simulink model "Noh_Nofusion"  (R2020b)
settings: Solver=FixedStepAuto  StartTime=0.0  StopTime=Inf  FixedStep=0.01  RelTol=1e-3
PostLoadFcn:
  | if any(exist('dsrtsu_mdlpostloadfcn', 'file') ~= 0), dsrtsu_mdlpostloadfcn('Execute', bdroot); end
InitFcn:
  | , if any(exist('rtifpga_mdlclblib', 'file') ~= 0), rtifpga_mdlclblib('Init', bdroot); end,
  | , if any(exist('dsmpb_private', 'file') ~= 0), dsmpb_private('dsmpb_mdlclblib', 'Init', bdroot); end,
undefined symbols (not defined in the file): ACC_TimeGap_DecSetSwt, ACC_TimeGap_IncSetSwt, AccelPedalPosn, AccelPedalPosnVldty, AccelPedlPosnDiagc, AccPedalOverride, ACU_ShiftInProgress, ADAS_Posn_CurLane, AESSwtReq, ALC_SwtReq, BrkPedalSts, CC_ACC_CANCEL_OFFSwt, CC_ACC_CRUISE_OFFSwt, CC_ACC_DecSetSpd_SetSwt, CC_ACC_IncSetSpd_ResuSwt, CC_ACCSwtErr, CharSpd_ms, CSA_NODE, CURRENT_GEAR, CurrentGearValid, DiscIntNeverNeededParam, DrvDoorSts, DrvSBR, DrvTrqReqOvld, ECMACCInterface, ECMRespACC, ELKSwtReq, EngLimpHomeSts, EngSpd, EngState, EngState_PHEV, EngTrqMaxActSpd, EngTrqMinAct, EPS_DrvInpTrqVal_HighReslolution, EPS_FailSts, EPS_LKATorqOvrlDlvd, EPS_LKATorqOvrlDlvdVld, EPS_LKATrqOvlDlvdSts, EPS_SteerMod, EPS_TrqSnsrSts, EQ4_APPINFO, EQ4_LA_ELEM, EQ4_LA_HDR, EQ4_LAP_ELEM, EQ4_LAP_HDR, EQ4_LH_ELEM, EQ4_LH_HDR, EQ4_LRE_ELEM, EQ4_LRE_HDR, ESS_PedSwtReq, ESS_VehSwtReq, FFogLmpSts_F_Pbox, FLWheelDriveDirection, FLWheelSpd, FrntWiprSwtSts, FrntWshrSwtSts, FRWheelDriveDirection, FRWheelSpd, HazardLmpSwtSts, HCU_AccelPedalPosn_Diag ... (+153)
libraries: simulink x132, dsmpblib x27
(part 9 of 14)

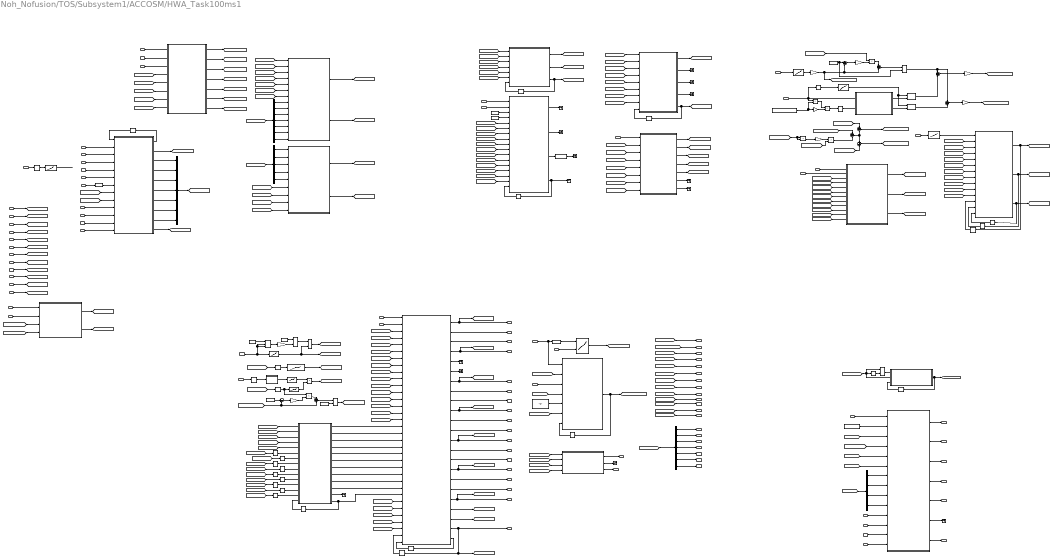
== system Noh_Nofusion/TOS/Subsystem1/ACCOSM/HWA_Task100ms1 ==
  note: EIA
  note: ASI_CalcPreOSF
  note: PLA
  note: ATS
  note: OTL
  ObjRange_m : Inport
  ObjDx_m : Inport  Port=2
  ObjDy_m : Inport  Port=3
  ObjValid : Inport  Port=4
  ObjClassification : Inport  Port=5
  ObjVxG_ms : Inport  Port=6
  ObjVyG_ms : Inport  Port=7
  ObjArG_ms2 : Inport  Port=8
  ObjWidth_m : Inport  Port=9
  ObjCnt : Inport  Port=10
  ObjMoveSts : Inport  Port=11
  ObjBrakeLightIndic : Inport  Port=12
  A2 : Inport  Port=13
  A1 : Inport  Port=14
  Conf : Inport  Port=15
  TimeGap : Inport  Port=16
  ACCMode : Inport  Port=17
  VxvRef_ms : Inport  Port=18
  kapCurvTraj : Inport  Port=19
  AlpSideSlipAngle : Inport  Port=20
  AlpWheelAngle : Inport  Port=21
  alpSumSlideCurveness : Inport  Port=22
  LongitudeAcc : Inport  Port=23
  TarLineValid : Inport  Port=24
  TarLine_A2 : Inport  Port=25
  TarLine_A1 : Inport  Port=26
  TarLine_A0 : Inport  Port=27
  1-D Lookup Table1 : Lookup_n-D  NumberOfTableDimensions=1  BreakpointsForDimension1=[0,8,23,55,60]  Table=[80,80,120,200,200]  RndMeth=Simplest  InputSameDT=on
  1-D Lookup Table2 : Lookup_n-D  NumberOfTableDimensions=1  BreakpointsForDimension1=[0,0.035,0.057,0.1]  Table=[1,1,0,0]  RndMeth=Simplest  InputSameDT=on
  ACCMode1 : InportShadow  Port=17
  ACC_DisplayBar : MATLAB Function  TreatAsAtomicUnit=on
  Abs : Abs
  Abs1 : Abs
  Abs2 : Abs
  AlpSideSlipAngle_1 : InportShadow  Port=20
  Bus Creator : BusCreator  Inputs=7
  Bus Selector : BusSelector  OutputSignals=dxC0,aPC0,bPC0,cPC0,aPC1,bPC1,cPC1
  Bus Selector1 : BusSelector  OutputSignals=dxC0,aPC0,bPC0,aPC1,bPC1
  Bus Selector2 : BusSelector  OutputSignals=dxC0,aPC0,bPC0,cPC0,aPC1,bPC1,cPC1
  Bus Selector3 : BusSelector  OutputSignals=dDeltaX,dDeltaY,CosOfPsi,SinOfPsi
  Compare To Constant : simulink/Logic and Bit Operations/Compare To Constant  relop=>=  const=1  OutDataTypeStr=boolean
  Compare To Constant1 : simulink/Logic and Bit Operations/Compare To Constant  relop=>=  const=0.7  OutDataTypeStr=boolean
  Constant : Constant  Value=15  OutDataTypeStr=single
  Constant1 : Constant  Value=0.6  OutDataTypeStr=single
  Constant3 : Constant  Value=[0.6,0.75,0.9;0.58,0.68,0.77;0.41,0.55,0.63;0.38,0.44,0.49]  OutDataTypeStr=single
  Constant6 : Constant  Value=0.1  OutDataTypeStr=single
  Data Type Conversion7 : DataTypeConversion  OutDataTypeStr=single
  DeltaDx : Lookup_n-D  NumberOfTableDimensions=1  BreakpointsForDimension1=[0,30,60,100,120,130]  Table=[2,4,6,8,9,9]  RndMeth=Simplest  InputSameDT=on
  DeltaDy : Lookup_n-D  NumberOfTableDimensions=1  BreakpointsForDimension1=[0,30,60,100,120,130]  Table=[0.5,0.5,1,1.2,1.5,1.5]  RndMeth=Simplest  InputSameDT=on
  DesireDistance : Lookup_n-D  BreakpointsForDimension1=[1,2,3,4]  BreakpointsForDimension2=[0,2.6,17,25,35,60]  BreakpointsForDimension1DataTypeStr=single  BreakpointsForDimension2DataTypeStr=single  Table=reshape([4,4.3,4.6,4.9,7.8,8.5,9,9.5,18,23,28,34,27,37,47,54,35,49,63,71,60,70,80,85],4,6)  TableDataTypeStr=single  RndMeth=Simplest
      settings: InputPortMap=u0,u1
  Dyc : MATLAB Function  TreatAsAtomicUnit=on
  DycCutIn : MATLAB Function  TreatAsAtomicUnit=on
  DycHistCalc : MATLAB Function  TreatAsAtomicUnit=on
  Fac : Lookup_n-D  NumberOfTableDimensions=1  BreakpointsForDimension1=[0,0.4,0.6,0.8]  Table=[1,1,1.5,1.5]  RndMeth=Simplest  InputSameDT=on
  Gain{,1,3..4} (4 alike) : Gain  Gain=0.5
  Gain2 : Gain  Gain=0.95
  Gain5 : Gain  Gain=0.02
  Gain6 : Gain  Gain=0.95
  Gain8 : Gain  Gain=0.02
  LostTargetCalc : MATLAB Function  TreatAsAtomicUnit=on
  Lpb : MATLAB Function  TreatAsAtomicUnit=on
  Memory{1..2,4,6,13..14} (6 alike) : Memory  InitialCondition=single(zeros(15,1))  InheritSampleTime=on
  Memory10 : Memory  InitialCondition=uint8(0)  InheritSampleTime=on
  Memory12 : Memory  InheritSampleTime=on
  Memory{8,15..16,18..22,25,27..28} (11 alike) : Memory  InitialCondition=single(0)  InheritSampleTime=on
  Memory17 : Memory  InitialCondition=uint8(0)  InheritSampleTime=on
  Memory24 : Memory  InitialCondition=false  InheritSampleTime=on
  Memory26 : Memory  InitialCondition=false  InheritSampleTime=on
  Memory3 : Memory  InheritSampleTime=on
  Memory30 : Memory  InitialCondition=uint8(0)  InheritSampleTime=on
  MinMax : MinMax  Function=max  Inputs=2
  MinMax1 : MinMax  Function=max  Inputs=2
  MinMax2 : MinMax  Inputs=2
  MinMax4 : MinMax  Inputs=2
  MinMax5 : MinMax  Function=max  Inputs=2
  MinMax6 : MinMax  Inputs=2
  OTL1 : Subsystem
  Plaus : MATLAB Function  TreatAsAtomicUnit=on
  Product{,1..6} (7 alike) : Product
  Product7 : Product  Inputs=/**
  Relational Operator1 : RelationalOperator  Operator===  OutDataTypeStr=boolean  RndMeth=Nearest
  Spw : MATLAB Function  TreatAsAtomicUnit=on
  Std : MATLAB Function  TreatAsAtomicUnit=on
  Sum1 : Sum  Inputs=|+-
  Sum10 : Sum  Inputs=-+
  Sum11 : Sum  Inputs=|+-
  Sum{2..4,13} (4 alike) : Sum
  Sum8 : Sum  Inputs=+-
  Sum9 : Sum  Inputs=+-
  Tapped Delay : simulink/Discrete/Tapped Delay  vinit=0.0  samptime=-1  NumDelays=4  DelayOrder=Newest  includeCurrent=on
  TarLineValid1 : InportShadow  Port=24
  TarLine_A0_1 : InportShadow  Port=27
  TarLine_A1_1 : InportShadow  Port=26
  TarLine_A2_1 : InportShadow  Port=25
  TargetBrake : MATLAB Function  TreatAsAtomicUnit=on
  TargetSelect : MATLAB Function  TreatAsAtomicUnit=on
  Terminator{,1,3,9..15,17..20} (14 alike) : Terminator
  TimeCalc : MATLAB Function  TreatAsAtomicUnit=on
  Trajectory : Subsystem  TreatAsAtomicUnit=on
  VxVy : Subsystem
  VxvRef_ms_{1..10} (10 alike) : InportShadow  Port=18
  VycCalc : MATLAB Function  TreatAsAtomicUnit=on
  alpSumSlideCurveness1 : InportShadow  Port=22
  dxMaxFollowPO : Lookup_n-D  NumberOfTableDimensions=1  BreakpointsForDimension1=[8.33,22.22,37.5]  Table=[90,120,120]  InternalRulePriority=Speed  RndMeth=Simplest  InputSameDT=on
  dyLaneWidthMin : Lookup_n-D  NumberOfTableDimensions=1  BreakpointsForDimension1=[0,2.78,8.33,10]  Table=[3,3,2.8,2.8]  InternalRulePriority=Speed  RndMeth=Simplest  InputSameDT=on
  dyLaneWidthMinHalfStatObj1 : Constant  Value=P_Global_DxvFrontBumper_m  OutDataTypeStr=single
  dyLaneWidthMinHalfStatObj10 : Constant  Value=2.2  OutDataTypeStr=single
  dyLaneWidthMinHalfStatObj2 : Constant  Value=2.2  OutDataTypeStr=single
  dyLaneWidthMinHalfStatObj5 : Constant  Value=0  OutDataTypeStr=single
  dyLaneWidthMinHalfStatObj7 : Constant  Value=0  OutDataTypeStr=single
  dyLaneWidthMinHalfStatObj9 : Constant  Value=2.2  OutDataTypeStr=single
  dyLaneWidthSteerAdapt : MATLAB Function  TreatAsAtomicUnit=on
  kapCurvTraj_{1..4} (4 alike) : InportShadow  Port=19
  t_dyLaneWidthSteerAdapt : Lookup_n-D  NumberOfTableDimensions=1  BreakpointsForDimension1=[0,0.02,0.05,0.1]  Table=[0,0,0.7,0.7]  InternalRulePriority=Speed  RndMeth=Simplest  InputSameDT=on
  wCutInVy : MATLAB Function  TreatAsAtomicUnit=on
  wCutOutVy : MATLAB Function  TreatAsAtomicUnit=on
  P0ID : Outport
  P2ID : Outport  Port=2
  P3ID : Outport  Port=3
  TargetBrake_b : Outport  Port=4
  P0Range : Outport  Port=5
  P0Vr : Outport  Port=6
  P2Vr : Outport  Port=7
  P3Vr : Outport  Port=8
  P0ArG : Outport  Port=9
  P2ArG : Outport  Port=10
  P3ArG : Outport  Port=11
  P0Dx : Outport  Port=12
  P2Dx : Outport  Port=13
  P3Dx : Outport  Port=14
  P0Dy : Outport  Port=15
  P2Dy : Outport  Port=16
  P3Dy : Outport  Port=17
  CutIn_b : Outport  Port=18
  TargetExist : Outport  Port=19
  DesireDis : Outport  Port=20
  Signal_ACC_TgtObjBarDisp : Outport  Port=21
  ObjDyc_m : Outport  Port=22
  ObjVy_ms : Outport  Port=23
  ObjVyc_ms : Outport  Port=24
  ObjSpw : Outport  Port=25
  ObjSpwLeft : Outport  Port=26
  ObjSpwRight : Outport  Port=27
  ObjPlaus : Outport  Port=28
  ObjPlausLeft : Outport  Port=29
  ObjPlausRight : Outport  Port=30
  ObjDycHist : Outport  Port=31
  ObjqDycHist : Outport  Port=32
  dxC0 : Outport  Port=33
  aPC0 : Outport  Port=34
  bPC0 : Outport  Port=35
  cPC0 : Outport  Port=36
  aPC1 : Outport  Port=37
  bPC1 : Outport  Port=38
  cPC1 : Outport  Port=39
  OTLValid : Outport  Port=40
  aOTL : Outport  Port=41
  bOTL : Outport  Port=42
  cOTL : Outport  Port=43
  dOTL : Outport  Port=44
  dxMaxOTL : Outport  Port=45
  TargetVyG : Outport  Port=46
  wires:
  TarLine_A0_1/1 -> OTL1/14(TarLineA0)
  TarLineValid1/1 -> OTL1/11(TarLineValid)
  TarLine_A1_1/1 -> OTL1/13(TarLineA1)
  TarLine_A2_1/1 -> OTL1/12(TarLineA2)
  Dyc/10(ObjDyc) -> [ObjDyc_m]
  DesireDistance/1 -> [DesireDistanceChar]
  Memory10/1 -> ACC_DisplayBar/7(DisplayBarK1)
  Constant3/1 -> ACC_DisplayBar/5(Scale)
  ACC_DisplayBar/1(DisplayBar) -> [Signal_ACC_TgtObjBarDisp], Memory10/1
  [TargetRange] -> ACC_DisplayBar/4(TargetRange)
  [TargetExist] -> ACC_DisplayBar/6(TargetExist)
  ACCMode/1 -> ACC_DisplayBar/3(ACCmode)
  TimeGap/1 -> ACC_DisplayBar/1(TimeGap), Data Type Conversion7/1
  VxvRef_ms_3/1 -> dyLaneWidthMin/1
  dyLaneWidthMin/1 -> Gain/1
  Gain/1 -> [dyLaneWidthMinHalf], Sum2/2, Sum1/2  "dyLaneWidthMinHalf"
  dyLaneWidthMinHalfStatObj1/1 -> Product/2, Gain3/1
  kapCurvTraj/1 -> Abs1/1, Product/1, dyLaneWidthSteerAdapt/1(kap)
  Product/1 -> Product1/1
  Gain3/1 -> Product1/2
  Product1/1 -> Abs/1
  Abs/1 -> dyLaneWidthSteerAdapt/2(dyAdapt)  "dyAdapt"
  Abs1/1 -> t_dyLaneWidthSteerAdapt/1
  t_dyLaneWidthSteerAdapt/1 -> MinMax1/1, MinMax/1
  dyLaneWidthSteerAdapt/1(dyLaneAdaptLeft) -> MinMax/2
  dyLaneWidthSteerAdapt/2(dyLaneAdaptRight) -> MinMax1/2
  MinMax/1 -> Sum3/2  "dyLaneWidthSteerAdaptLeft"
  MinMax1/1 -> Sum4/2  "dyLaneWidthSteerAdaptRight"
  Sum1/1 -> Gain5/1
  Gain5/1 -> Product2/2
  [ObjDx_m] -> Product2/1
  Product2/1 -> Sum2/1
  Sum2/1 -> MinMax2/1
  dyLaneWidthMinHalfStatObj2/1 -> MinMax2/2, Sum1/1
  MinMax2/1 -> Sum3/1, Sum4/1
  Sum3/1 -> Gain2/1
  VxvRef_ms_5/1 -> VxVy/1(VxvRef)
  VxVy/1(Vx) -> [ObjVx_ms]
  VxVy/2(Vy) -> [ObjVy_ms]
  [ObjVyG_ms] -> VxVy/4(VyG)
  [ObjVxG_ms] -> VxVy/3(VxG)
  kapCurvTraj_3/1 -> VxVy/2(Kap)
  kapCurvTraj_2/1 -> Trajectory/1(Kap)
  AlpSideSlipAngle/1 -> Trajectory/3(AlpSideSlipAngle)
  VxvRef_ms_6/1 -> Trajectory/2(VxvRef)
  [ObjValid] -> Trajectory/4(ObjValid)
  [ObjCnt] -> Trajectory/8(ObjCntAlive)
  [ObjDx_m] -> Trajectory/5(ObjDx)
  [ObjDy_m] -> Trajectory/6(ObjDy)
  [ObjMoveSts] -> Trajectory/7(ObjClass)
  Memory8/1 -> Dyc/1(kapTrajFiltK1)
  Dyc/1(kapTrajFilt) -> Memory8/1
  AlpSideSlipAngle_1/1 -> Dyc/4(alpSideSlipAngle)
  kapCurvTraj_1/1 -> Dyc/3(kapTraj)
  ObjDx_m/1 -> [ObjDx_m]
  Compare To Constant/1 -> Dyc/7(LineValid)
  VxvRef_ms_7/1 -> Dyc/2(vRef)
  1-D Lookup Table2/1 -> ?  "AlpWheelAngleFactor"
  Abs2/1 -> 1-D Lookup Table2/1
  AlpWheelAngle/1 -> Abs2/1
  ObjRange_m/1 -> [ObjRange_m]
  ObjMoveSts/1 -> [ObjMoveSts]
  ObjVxG_ms/1 -> [ObjVxG_ms]
  ObjWidth_m/1 -> [ObjWidth_m]
  ObjClassification/1 -> [ObjClassification]
  ObjArG_ms2/1 -> [ObjArG_ms2]
  Conf/1 -> Compare To Constant/1
  ObjDy_m/1 -> [ObjDy_m]
  ObjCnt/1 -> [ObjCnt]
  ObjVyG_ms/1 -> [ObjVyG_ms]
  [ObjDy_m] -> Dyc/9(ObjDy)
  [ObjDx_m] -> Dyc/8(ObjDx)
  Dyc/9(cPC1) -> Bus Creator/7
  Dyc/7(aPC1) -> Bus Creator/5
  Dyc/8(bPC1) -> Bus Creator/6
  ObjValid/1 -> [ObjValid]
  Dyc/4(aPC0) -> Bus Creator/2
  Dyc/5(bPC0) -> Bus Creator/3
  Dyc/6(cPC0) -> Bus Creator/4
  Dyc/3(dxC0) -> Bus Creator/1
  Data Type Conversion7/1 -> DesireDistance/1
  Sum4/1 -> Gain6/1
  Bus Creator/1 -> [EgoLine]
  [ObjValid] -> DycHistCalc/7(ObjValid)
  DycHistCalc/1(ObjDycHist) -> [ObjDycHist]
  DycHistCalc/2(ObjqDycHist) -> [ObjqDycHist]
  [ObjValid] -> VycCalc/6(ObjValid)
  [ObjDx_m] -> VycCalc/7(ObjDx)
  [ObjVxG_ms] -> VycCalc/8(ObjVxG)
  [ObjVyG_ms] -> VycCalc/9(ObjVyG)
  VycCalc/1(ObjVyc) -> [ObjVyc]
  [EgoLine] -> Bus Selector/1
  Bus Selector/4 -> DycHistCalc/11(cP0)  "<cPC0>"
  Bus Selector/3 -> DycHistCalc/10(bP0)  "<bPC0>"
  Bus Selector/5 -> DycHistCalc/12(aP1)  "<aPC1>"
  Bus Selector/2 -> DycHistCalc/9(aP0)  "<aPC0>"
  Bus Selector/6 -> DycHistCalc/13(bP1)  "<bPC1>"
  Bus Selector/1 -> DycHistCalc/8(dxC0)  "<dxC0>"
  Bus Selector/7 -> DycHistCalc/14(cP1)  "<cPC1>"
  [EgoLine] -> Bus Selector1/1
  Bus Selector1/3 -> VycCalc/3(bP0)  "<bPC0>"
  Bus Selector1/2 -> VycCalc/2(aP0)  "<aPC0>"
  Bus Selector1/4 -> VycCalc/4(aP1)  "<aPC1>"
  Bus Selector1/1 -> VycCalc/1(dxC0)  "<dxC0>"
  Bus Selector1/5 -> VycCalc/5(bP1)  "<bPC1>"
  Dyc/2(kapCourseErr) -> [kapCourseErr]
  [ObjDx_m] -> Product3/2, Product3/1
  Product3/1 -> Gain4/1
  Gain4/1 -> Product4/1
  [kapCourseErr] -> Product4/2
  Product4/1 -> Sum8/2
  [dyLaneWidthMinHalf] -> Sum8/1
  [dyLaneWidthRight] -> Sum9/1
  Sum8/1 -> Sum9/2, Sum10/1
  Sum9/1 -> [dyEdgeWidthRight]  "dyEdgeWidthRight"
  [dyLaneWidthLeft] -> Sum10/2
  Sum10/1 -> [dyEdgeWidthLeft]  "dyEdgeWidthLeft"
  VycCalc/2(ObjYawAngle) -> [ObjYawAngle]
  VxvRef_ms_1/1 -> Lpb/1(vRef)
  alpSumSlideCurveness/1 -> Lpb/2(alpSumSlideCurveness)
  [ObjValid] -> Lpb/3(ObjValid)
  [ObjDyc_m] -> Lpb/4(ObjDyc)
  [ObjDycHist] -> Lpb/5(ObjDycHist)
  [ObjqDycHist] -> Lpb/6(ObjqDycHist)
  [ObjVyc] -> Lpb/7(ObjVyc)
  [ObjYawAngle] -> Lpb/8(ObjYawAngle)
  Lpb/1(ObjLpb) -> [ObjLpb]
  Lpb/2(ObjLpbL) -> [ObjLpbLeft]
  Lpb/3(ObjLpbR) -> [ObjLpbRight]
  [dyLaneWidthRight] -> Lpb/9(ObjDylaneEdgeRight)
  [dyEdgeWidthLeft] -> Lpb/12(ObjDyEdgeWidthLeft)
  [dyEdgeWidthRight] -> Lpb/10(ObjDyEdgeWidthRight)
  [dyLaneWidthLeft] -> Lpb/11(ObjDylaneEdgeLeft)
  [ObjValid] -> DycCutIn/1(ObjValid)
  [ObjDyc_m] -> DycCutIn/2(ObjDyc)
  [ObjMoveSts] -> DycCutIn/3(ObjMoveSts)
  [ObjCnt] -> DycCutIn/4(ObjCnt)
  [ObjDycHist] -> DycCutIn/5(ObjDycHist)
  [ObjqDycHist] -> DycCutIn/6(ObjqDycHist)
  DycCutIn/3(ObjDycFilt) -> [ObjDycFilt], Memory1/1
  DycCutIn/1(ObjDycCutIn) -> [ObjDycCutIn]
  Memory1/1 -> DycCutIn/7(dycFiltK1)
  DycCutIn/2(ObjMove_b) -> [ObjDrive_b]
  [ObjValid] -> wCutOutVy/5(ObjValid)
  [ObjDycCutIn] -> wCutOutVy/6(ObjDycCutIn)
  [ObjWidth_m] -> wCutOutVy/7(ObjWidth)
  [ObjVyc] -> wCutOutVy/8(ObjVyc)
  [ObjDx_m] -> wCutOutVy/9(ObjDx)
  [ObjDycFilt] -> wCutOutVy/16(ObjDycFilt)
  wCutOutVy/4(ObjwCutoutVy) -> Terminator17/1, Memory2/1
  Memory2/1 -> wCutOutVy/17(ObjwCutoutVyK1)
  wCutOutVy/1(ObjtPrediction4CutOut) -> Terminator14/1
  wCutOutVy/2(ObjDycCutOutPredict) -> Terminator15/1
  kapCurvTraj_4/1 -> wCutOutVy/2(kap)
  VxvRef_ms_8/1 -> wCutOutVy/1(vRef)
  dyLaneWidthMinHalfStatObj5/1 -> wCutOutVy/3(tDirIndLeft)
  dyLaneWidthMinHalfStatObj7/1 -> wCutOutVy/4(tDirIndRight)
  [ObjDy_m] -> wCutOutVy/10(ObjDy)
  [ObjVx_ms] -> wCutOutVy/11(ObjVx)
  [ObjVy_ms] -> wCutOutVy/12(ObjVy)
  [ObjDyc_m] -> wCutOutVy/13(ObjDyc)
  [ObjDrive_b] -> wCutOutVy/14(ObjDrive_b)
  [ObjCnt] -> wCutOutVy/15(ObjCnt)
  wCutOutVy/3(ObjwCutOutTurnOff) -> Compare To Constant1/1
  [ObjValid] -> wCutInVy/1(ObjValid)
  [ObjDycCutIn] -> wCutInVy/2(ObjDycCutIn)
  [ObjWidth_m] -> wCutInVy/3(ObjWidth)
  [ObjVyc] -> wCutInVy/4(ObjVyc)
  [ObjDx_m] -> wCutInVy/5(ObjDx)
  [ObjDy_m] -> wCutInVy/6(ObjDy)
  [ObjCnt] -> wCutInVy/7(ObjCnt)
  [ObjDycFilt] -> wCutInVy/8(ObjDycFilt)
  wCutInVy/5(ObjwCutInVy) -> [ObjwCutIn], Memory4/1
  Memory4/1 -> wCutInVy/9(ObjwCutInVyK1)
  wCutInVy/2(ObjtPrediction4CutIn) -> Terminator18/1
  wCutInVy/3(ObjDycCutInPredict) -> Terminator19/1
  wCutInVy/1(DycASI) -> [DycASI]
  alpSumSlideCurveness1/1 -> Spw/1(AlpSumSlideCurveness)
  [kapCourseErr] -> Spw/2(kapCourseErr)
  [ObjValid] -> Spw/3(ObjValid)
  [DycASI] -> Spw/4(DycASI)
  [ObjDx_m] -> Spw/5(ObjDx)
  Spw/1(ObjSpw) -> [ObjSpw]
  Spw/2(ObjSpwLeft) -> [ObjSpwLeft]
  Spw/3(ObjSpwRight) -> [ObjSpwRight]
  wCutInVy/4(ObjCutIn_b) -> Terminator20/1
  Spw/4(ObjOnLeft) -> [ObjOnLeft]
  Spw/5(ObjOnRight) -> [ObjOnRight]
  [ObjDyc_m] -> Spw/6(ObjDyc)
  [ObjDycHist] -> Spw/7(ObjDycHist)
  [ObjqDycHist] -> Spw/8(ObjqDycHist)
  Plaus/3(ObjPlausRight) -> Memory6/1, [ObjPlausRight]
  Plaus/2(ObjPlausLeft) -> [ObjPlausLeft], Memory13/1
  Plaus/1(ObjPlaus) -> [ObjPlaus], Memory14/1
  dxMaxFollowPO/1 -> Plaus/1(dxMaxFollow)
  VxvRef_ms_9/1 -> dxMaxFollowPO/1
  [ObjValid] -> Plaus/2(ObjValid)
  [ObjDx_m] -> Plaus/3(ObjDx)
  [ObjVx_ms] -> Plaus/4(ObjVx)
  [ObjOnLeft] -> Plaus/5(ObjOnLeft)
  [ObjOnRight] -> Plaus/6(ObjOnRight)
  [ObjDycHist] -> Plaus/7(ObjDycHist)
  [ObjqDycHist] -> Plaus/8(ObjqDycHist)
  [ObjLpb] -> Plaus/9(ObjLpb)
  [ObjLpbLeft] -> Plaus/10(ObjLpbLeft)
  [ObjLpbRight] -> Plaus/11(ObjLpbRight)
  Memory6/1 -> Plaus/14(ObjPlausRightK1)
  Memory13/1 -> Plaus/13(ObjPlausLeftK1)
  Memory14/1 -> Plaus/12(ObjPlausK1)
  [ObjDx_m] -> TargetSelect/6(Dx)
  TargetSelect/12(P3ArG) -> P3ArG/1
  TargetSelect/9(P3Vr) -> P3Vr/1
  [ObjDyc_m] -> ObjDyc_m/1
  TargetSelect/17(P2Dy) -> P2Dy/1
  TargetSelect/11(P2ArG) -> P2ArG/1
  [ObjMoveSts] -> TargetSelect/30(MoveSts)
  [ObjArG_ms2] -> TargetSelect/8(ArG)
  TargetSelect/18(P3Dy) -> P3Dy/1
  TargetSelect/8(P2Vr) -> P2Vr/1
  [ObjClassification] -> TargetSelect/29(Classfication)
  [ObjValid] -> TargetSelect/3(Valid)
  TargetSelect/3(P3ID) -> P3ID/1
  VxvRef_ms/1 -> TargetSelect/2(vRef)
  ACCMode1/1 -> TargetSelect/1(ACCmode)
  [TarLimDx] -> TargetSelect/31(TarLimDx)
  Memory24/1 -> TargetSelect/33(TargetExistK1)
  TargetSelect/4(P0Range) -> P0Range/1, [TargetRange]
  TargetSelect/15(P3Dx) -> P3Dx/1
  [ObjRange_m] -> TargetSelect/4(Range)
  [ObjVx_ms] -> TargetSelect/5(Vr)
  [Signal_ACC_TgtObjBarDisp] -> Signal_ACC_TgtObjBarDisp/1
  [ObjSpwRight] -> TargetSelect/16(spwRight)
  TargetSelect/2(P2ID) -> P2ID/1
  [ObjVy_ms] -> ObjVy_ms/1
  [ObjDy_m] -> TargetSelect/7(Dy)
  TargetSelect/13(P0Dx) -> [TargetDx], P0Dx/1
  TargetSelect/7(P0Vr) -> [TargetVr], P0Vr/1
  [DesireDistanceChar] -> DesireDis/1  "DesireDis"
  TargetSelect/19(TargetCutIn_b) -> [TargetCutIn_b], CutIn_b/1
  TargetSelect/22(TargetExist) -> Memory24/1, [TargetExist], TargetExist/1
  TargetSelect/10(P0ArG) -> [TargetArG], P0ArG/1
  TargetSelect/14(P2Dx) -> P2Dx/1
  TargetSelect/16(P0Dy) -> [TargetDy], P0Dy/1
  [ObjPlaus] -> TargetSelect/12(plaus)
  [ObjwCutIn] -> TargetSelect/13(wCutIn)
  [ObjSpw] -> TargetSelect/14(spw)
  [ObjSpwLeft] -> TargetSelect/15(spwLeft)
  MinMax4/1 -> [dyLaneWidth]
  LostTargetCalc/12(tTargetLost) -> Memory27/1, TargetSelect/27(tTargetLost)
  [ObjValid] -> LostTargetCalc/1(ObjValid)
  [ObjDx_m] -> LostTargetCalc/2(ObjDx)
  [ObjDy_m] -> LostTargetCalc/3(ObjDy)
  TargetSelect/20(P0Dyc) -> [TargetDyc]
  TargetSelect/21(P0Vyc) -> [TargetVyc]
  [TargetID] -> Memory17/1
  Memory17/1 -> LostTargetCalc/6(P0IDK1)
  [TargetVr] -> Memory18/1
  Memory18/1 -> LostTargetCalc/7(P0VxK1)
  Memory20/1 -> LostTargetCalc/8(P0DxK1)
  Memory21/1 -> LostTargetCalc/9(P0DyK1)
  Memory22/1 -> LostTargetCalc/12(P0DycK1)
  Memory25/1 -> LostTargetCalc/13(P0VycK1)
  Memory26/1 -> LostTargetCalc/14(P0CutIn_bK1)
  Memory27/1 -> LostTargetCalc/15(tTargetLostK1)
  [TargetDx] -> Memory20/1
  [TargetDy] -> Memory21/1
  [TargetDyc] -> Memory22/1
  [TargetVyc] -> Memory25/1
  [TargetCutIn_b] -> Memory26/1
  [ObjVyc] -> TargetSelect/10(Vyc)
  [ObjDyc_m] -> TargetSelect/9(Dyc)
  dyLaneWidthMinHalfStatObj9/1 -> Sum11/1
  Sum11/1 -> Gain8/1
  Gain8/1 -> Product6/2
  Sum13/1 -> MinMax4/1
  Product6/1 -> Sum13/1
  [dyLaneWidthMinHalf] -> Sum13/2, Sum11/2  "dyLaneWidthMinHalf"
  Memory19/1 -> LostTargetCalc/10(P0RangeK1)
  [TargetRange] -> Memory19/1
  Memory28/1 -> LostTargetCalc/11(P0ArGK1)
  [TargetArG] -> Memory28/1
  Memory15/1 -> Product6/1, DeltaDx/1
  TargetSelect/1(P0ID) -> P0ID/1, [TargetID]
  TargetSelect/23(TargetReplacedCnt) -> Memory30/1
  Memory30/1 -> TargetSelect/34(TargetReplacedCntK1)
  DeltaDy/1 -> [DeltaDy]
  Memory16/1 -> DeltaDy/1
  [TargetDy] -> Memory16/1
  Product5/1 -> [DeltaDx]
  DeltaDx/1 -> Product5/2
  LongitudeAcc/1 -> Tapped Delay/1
  [TargetDx] -> Memory15/1
  Std/1(y) -> Fac/1
  Fac/1 -> Product5/1
  Tapped Delay/1 -> Std/1(u)
  [DesireDistanceChar] -> ACC_DisplayBar/2(DesireDistance)
  [DeltaDx] -> LostTargetCalc/4(DeltaDx)
  [DeltaDy] -> LostTargetCalc/5(DeltaDy)
  dyLaneWidthMinHalfStatObj10/1 -> MinMax4/2
  LostTargetCalc/1(ReID) -> TargetSelect/17(ReID)
  LostTargetCalc/2(ReRange) -> TargetSelect/18(ReRange)
  LostTargetCalc/3(ReArG) -> TargetSelect/19(ReArG)
  LostTargetCalc/4(ReDx) -> TargetSelect/20(ReDx)
  LostTargetCalc/5(ReDy) -> TargetSelect/21(ReDy)
  LostTargetCalc/6(ReVx) -> TargetSelect/22(ReVx)
  LostTargetCalc/7(ReCutIn_b) -> TargetSelect/23(ReCutIn_b)
  LostTargetCalc/8(ReDyc) -> TargetSelect/24(ReDyc)
  LostTargetCalc/9(ReVyc) -> TargetSelect/25(ReVyc)
  LostTargetCalc/10(TargetLost_b) -> TargetSelect/26(TargetLost_b)
  [dyLaneWidth] -> TargetSelect/28(dyLaneWidth)
  LostTargetCalc/11(Covered_b) -> Terminator9/1
  [ObjVyc] -> ObjVyc_ms/1
  [ObjSpw] -> ObjSpw/1
  [ObjSpwLeft] -> ObjSpwLeft/1
  [ObjSpwRight] -> ObjSpwRight/1
  [ObjPlaus] -> ObjPlaus/1
  [ObjPlausLeft] -> ObjPlausLeft/1
  [ObjPlausRight] -> ObjPlausRight/1
  TargetSelect/5(P2Range) -> Terminator10/1
  TargetSelect/6(P3Range) -> Terminator11/1
  [EgoLine] -> Bus Selector2/1
  Bus Selector2/1 -> dxC0/1  "<dxC0>"
  Bus Selector2/2 -> aPC0/1  "<aPC0>"
  Bus Selector2/3 -> bPC0/1  "<bPC0>"
  Bus Selector2/4 -> cPC0/1  "<cPC0>"
  Bus Selector2/5 -> aPC1/1  "<aPC1>"
  Bus Selector2/6 -> bPC1/1  "<bPC1>"
  Bus Selector2/7 -> cPC1/1  "<cPC1>"
  Spw/6(ObjDycASI) -> Terminator12/1
  Spw/7(ObjDyKapErr) -> Terminator13/1
  [ObjqDycHist] -> ObjqDycHist/1
  [ObjDycHist] -> ObjDycHist/1
  A2/1 -> Dyc/5(A2)
  A1/1 -> Dyc/6(A1)
  [TargetID] -> TargetBrake/1(ID)
  [ObjBrakeLightIndic] -> TargetBrake/4(BrakeLightIndic)
  ObjBrakeLightIndic/1 -> [ObjBrakeLightIndic]
  TargetBrake/1(TargetBrake_b) -> TargetBrake_b/1
  VxvRef_ms_2/1 -> DesireDistance/2
  Constant/1 -> MinMax5/1
  VxvRef_ms_4/1 -> Product7/2, Product7/3, 1-D Lookup Table1/1
  1-D Lookup Table1/1 -> MinMax6/2, [TarLimDx]
  Gain1/1 -> MinMax5/2
  Product7/1 -> Gain1/1
  MinMax5/1 -> MinMax6/1
  [TarLimS0Dx] -> TargetSelect/32(TarLimS0Dx)
  Constant1/1 -> Product7/1
  MinMax6/1 -> [TarLimS0Dx]
  [ObjCnt] -> TargetSelect/11(Cnt)
  Trajectory/1(Out8) -> [TrajHistBufferBTrajEnd]
  Trajectory/2(Out9) -> [ObjTrajNumber]
  Trajectory/3(Out10) -> [TrajCurrentIndex]
  Trajectory/4(Out11) -> [TrajHistBufferBValid]
  Trajectory/5(Out12) -> [TrajHistBufferDxv]
  Trajectory/6(Out13) -> [TrajHistBufferDyv]
  [TrajHistBufferBTrajEnd] -> DycHistCalc/1(TrajHistBufferBTrajEnd)
  [ObjTrajNumber] -> DycHistCalc/2(ObjTrajNumber)
  [TrajCurrentIndex] -> DycHistCalc/3(TrajCurrentIndex)
  [TrajHistBufferBValid] -> DycHistCalc/4(TrajHistBufferBValid)
  [TrajHistBufferDxv] -> DycHistCalc/5(TrajHistBufferDxv)
  [TrajHistBufferDyv] -> DycHistCalc/6(TrajHistBufferDyv)
  TarLine_A1/1 -> Dyc/12(TarLineA1)
  TarLineValid/1 -> Dyc/10(TarLineValid)
  TarLine_A2/1 -> Dyc/11(TarLineA2)
  Compare To Constant1/1 -> Terminator1/1
  [ObjVyG_ms] -> TargetBrake/3(VyG)
  TargetBrake/3(TargetVyG) -> TargetVyG/1
  [ObjVxG_ms] -> TargetBrake/2(VxG)
  TargetBrake/2(TargetVxG) -> Terminator3/1
  [TargetID] -> TimeCalc/2(TargetID), Relational Operator1/1, Memory12/1
  Relational Operator1/1 -> TimeCalc/1(SameTarget)
  TimeCalc/1(tSameHandleT) -> Memory3/1, [tSameHandleT1]
  Memory3/1 -> TimeCalc/3(tSameHandleTK1)
  Memory12/1 -> Relational Operator1/2
  Trajectory/7(EgoMove) -> [EgoMove]
  Constant6/1 -> OTL1/2(tCycle)
  Bus Selector3/2 -> OTL1/8(EgoDDeltaY)  "<dDeltaY>"
  Bus Selector3/4 -> OTL1/10(EgoSinOfPsi)  "<SinOfPsi>"
  [TargetDy] -> OTL1/6(P0Dy)
  [tSameHandleT1] -> OTL1/3(tSameHandle)
  Bus Selector3/3 -> OTL1/9(EgoCosOfPsi)  "<CosOfPsi>"
  Bus Selector3/1 -> OTL1/7(EgoDDeltaX)  "<dDeltaX>"
  [TargetDx] -> OTL1/5(P0Dx)
  [EgoMove] -> Bus Selector3/1
  OTL1/1(LineValid) -> OTLValid/1
  OTL1/2(a) -> aOTL/1
  OTL1/3(b) -> bOTL/1
  OTL1/4(c) -> cOTL/1
  OTL1/5(d) -> dOTL/1
  OTL1/7(dxMax) -> dxMaxOTL/1
  OTL1/6(dxMin) -> Terminator/1
  TarLine_A0/1 -> Dyc/13(TarLineA0)
  Gain2/1 -> [dyLaneWidthLeft]
  Gain6/1 -> [dyLaneWidthRight]
  [TargetCutIn_b] -> OTL1/4(CutIn)
  VxvRef_ms_10/1 -> OTL1/1(vRef)

== system Noh_Nofusion/TOS/Subsystem1/ACCOSM/ObjMatrixTransit ==
  EQ4_OBJ : Inport
  Bus Creator : BusCreator  Inputs=14
  Bus Selector4 : BusSelector  OutputSignals=EQ4_OBJ_HDR.OBJ_Sync_ID,EQ4_OBJ_HDR.OBJ_VRU_Count,EQ4_OBJ_HDR.OBJ_VD_Count,EQ4_OBJ_HDR.OBJ_General_OBJ_Count,EQ4_OBJ_HDR.OBJ_Animal_Count,EQ4_OBJ_ELEM
  Data Type Conversion : DataTypeConversion
  IFV2FrontBumper : Constant  Value=1.7  OutDataTypeStr=single
  IFV2RearAxis : Constant  Value=2.1  OutDataTypeStr=single
  Subsystem : Subsystem
  Sum : Sum  Inputs=++++
  Sum1 : Sum  Inputs=|-+
  Sum5 : Sum  Inputs=++|
  Terminator1 : Terminator
  VisObjSts : Outport
  wires:
  Subsystem/6(ObjLatVel) -> Bus Creator/7  "ObjLatVel"
  Subsystem/4(ObjClassification) -> Bus Creator/5  "ObjClassification"
  Subsystem/2(ObjValid) -> Bus Creator/3  "ObjValid"
  Subsystem/7(ObjLongAccel) -> Bus Creator/8  "ObjLongAccel"
  Subsystem/5(ObjLatPos) -> Bus Creator/6  "ObjLatPos"
  Subsystem/3(ObjBrakeLightIndic) -> Bus Creator/4  "ObjBrakeLightIndic"
  Subsystem/9(ObjWidth) -> Bus Creator/10  "ObjWidth"
  Subsystem/12(ObjLongPos) -> Sum1/2, Sum5/1
  Subsystem/8(ObjLongVel) -> Bus Creator/9  "ObjLongVel"
  Subsystem/10(ObjCnt) -> Bus Creator/11  "ObjCnt"
  Sum1/1 -> Bus Creator/13  "ObjRange_m"
  Subsystem/11(ObjMoveSts) -> Bus Creator/12  "ObjMoveSts"
  Sum5/1 -> Bus Creator/14  "ObjDx_m"
  IFV2RearAxis/1 -> Sum5/2
  Data Type Conversion/1 -> Bus Creator/1  "Cnt"
  IFV2FrontBumper/1 -> Sum1/1
  Bus Creator/1 -> VisObjSts/1  "ObjSts"
  Subsystem/1(ObjID) -> Bus Creator/2  "ObjID"
  Bus Selector4/6 -> Subsystem/2(<EQ4_OBJ_ELEM>)  "<EQ4_OBJ_ELEM>"
  Sum/1 -> Subsystem/1(Count)
  Bus Selector4/4 -> Sum/3  "<OBJ_General_OBJ_Count>"
  Bus Selector4/3 -> Sum/2  "<OBJ_VD_Count>"
  Bus Selector4/2 -> Sum/1  "<OBJ_VRU_Count>"
  Bus Selector4/1 -> Data Type Conversion/1  "<OBJ_Sync_ID>"
  Bus Selector4/5 -> Sum/4  "<OBJ_Animal_Count>"
  EQ4_OBJ/1 -> Bus Selector4/1
  Subsystem/13(P) -> Terminator1/1

== system Noh_Nofusion/TOS/Subsystem1/ACCOSM/rollingcounter 1 ==
  Constant7 : Constant  OutDataTypeStr=Inherit: Inherit via back propagation
  Constant8 : Constant  Value=7  OutDataTypeStr=Inherit: Inherit via back propagation
  Constant9 : Constant  Value=0  OutDataTypeStr=Inherit: Inherit via back propagation
  Relational Operator : RelationalOperator  Operator=>  OutDataTypeStr=boolean  RndMeth=Nearest
  Sum : Sum  Inputs=|++
  Switch : Switch  Criteria=u2 ~= 0  Threshold=1
  Unit Delay : UnitDelay  SampleTime=-1  HasFrameUpgradeWarning=on
  cnt : Outport
  wires:
  Constant9/1 -> Switch/1
  Sum/1 -> Switch/3, Relational Operator/1
  Constant8/1 -> Relational Operator/2
  Unit Delay/1 -> Sum/2
  Constant7/1 -> Sum/1
  Relational Operator/1 -> Switch/2
  Switch/1 -> cnt/1, Unit Delay/1

== system Noh_Nofusion/Common1/Subsystem7/DS/DriverStsConditnJudge/DSGoodUnbeliv2LowDistractnJudge ==
  note: %Note
      | Conditions of distraction state from Good∥Unbelievable to Low as follow:
      | DMSSts_ACC is 0x02: Active
      | && HeadDetn is 0x01: Yes
      | && DistrctnLevel_ACC is 0x01: Low level distraction
      | && DistrctnQlty_ACC≥ 85%
      | && During time≥1s(adjustable)
  canDMSSts : Inport
  canHeadDetn : Inport  Port=2
  canDistrctnLevel : Inport  Port=3
  canDistrctnQlty : Inport  Port=4
  PtDSGoodUnbeliv2LowDistrctn : Inport  Port=5
  Compare To Constant : simulink/Logic and Bit Operations/Compare To Constant  relop===  const=2  OutDataTypeStr=boolean
  Compare To Constant1 : simulink/Logic and Bit Operations/Compare To Constant  relop===  const=1  OutDataTypeStr=boolean
  Compare To Constant2 : simulink/Logic and Bit Operations/Compare To Constant  relop===  const=1  OutDataTypeStr=boolean
  Compare To Constant4 : simulink/Logic and Bit Operations/Compare To Constant  relop=>=  const=85  OutDataTypeStr=boolean
  Compare To Constant8 : simulink/Logic and Bit Operations/Compare To Constant  relop=<=  const=100  OutDataTypeStr=boolean
  Data Type Conversion : DataTypeConversion  OutDataTypeStr=single
  Logical Operator : Logic  Inputs=5  AllPortsSameDT=off  OutDataTypeStr=boolean
  Relational Operator : RelationalOperator  OutDataTypeStr=boolean  RndMeth=Simplest
  counter : DiscreteIntegrator  ExternalReset=either  SampleTime=-1  LimitOutput=on  UpperSaturationLimit=10  LowerSaturationLimit=-10  ICPrevOutput=DiscIntNeverNeededParam  ICPrevScaledInput=DiscIntNeverNeededParam
  DSGoodUnbeliv2LowDistractn : Outport
  wires:
  Data Type Conversion/1 -> counter/1, counter/2
  PtDSGoodUnbeliv2LowDistrctn/1 -> Relational Operator/2
  Relational Operator/1 -> DSGoodUnbeliv2LowDistractn/1
  Compare To Constant8/1 -> Logical Operator/5
  Compare To Constant4/1 -> Logical Operator/4
  Compare To Constant2/1 -> Logical Operator/3
  Compare To Constant/1 -> Logical Operator/1
  Compare To Constant1/1 -> Logical Operator/2
  canDistrctnQlty/1 -> Compare To Constant4/1, Compare To Constant8/1
  counter/1 -> Relational Operator/1
  Logical Operator/1 -> Data Type Conversion/1
  canDistrctnLevel/1 -> Compare To Constant2/1
  canHeadDetn/1 -> Compare To Constant1/1
  canDMSSts/1 -> Compare To Constant/1

== system Noh_Nofusion/Common1/Subsystem7/DS/DriverStsConditnJudge/DSGoodUnbeliv2LowDrowsnsJudge ==
  note: %Note
      | Conditions of drowsns state from Good∥Unbelievable to Low as follow:
      | DMSSts_ACC is 0x02: Active
      | && HeadDetn is 0x01: Yes
      | && DrowsnsLevel_ACC is 0x1: Low level Drowsiness
      | && DrowsnsQlty_ACC≥85%
      | && During time≥3s(adjustable)
  canDMSSts : Inport
  canHeadDetn : Inport  Port=2
  canDrowsnsLevel : Inport  Port=3
  PtDSGoodUnbeliv2LowDrowsns : Inport  Port=4
  Compare To Constant : simulink/Logic and Bit Operations/Compare To Constant  relop===  const=2  OutDataTypeStr=boolean
  Compare To Constant1 : simulink/Logic and Bit Operations/Compare To Constant  relop===  const=1  OutDataTypeStr=boolean
  Compare To Constant2 : simulink/Logic and Bit Operations/Compare To Constant  relop===  const=1  OutDataTypeStr=boolean
  Data Type Conversion : DataTypeConversion  OutDataTypeStr=single
  Logical Operator : Logic  Inputs=3  AllPortsSameDT=off  OutDataTypeStr=boolean
  Relational Operator : RelationalOperator  OutDataTypeStr=boolean  RndMeth=Simplest
  counter : DiscreteIntegrator  ExternalReset=either  SampleTime=-1  LimitOutput=on  UpperSaturationLimit=10  LowerSaturationLimit=-10  ICPrevOutput=DiscIntNeverNeededParam  ICPrevScaledInput=DiscIntNeverNeededParam
  DSGoodUnbeliv2LowDrowsns : Outport
  wires:
  Data Type Conversion/1 -> counter/2, counter/1
  PtDSGoodUnbeliv2LowDrowsns/1 -> Relational Operator/2
  canDMSSts/1 -> Compare To Constant/1
  canHeadDetn/1 -> Compare To Constant1/1
  canDrowsnsLevel/1 -> Compare To Constant2/1
  Logical Operator/1 -> Data Type Conversion/1
  counter/1 -> Relational Operator/1
  Compare To Constant1/1 -> Logical Operator/2
  Compare To Constant/1 -> Logical Operator/1
  Compare To Constant2/1 -> Logical Operator/3
  Relational Operator/1 -> DSGoodUnbeliv2LowDrowsns/1

== system Noh_Nofusion/Common1/Subsystem7/DS/DriverStsConditnJudge/DSGoodUnbeliv2MidDistractnJudge ==
  note: %Note
      | Conditions of distraction state from Good∥Unbelievable to Middle as follow:
      | DMSSts_ACC is 0x02: Active
      | && HeadDetn is 0x01: Yes
      | && DistrctnLevel_ACC is 0x02: Middle level distraction
      | && DistrctnQlty_ACC≥ 85%
      | && During time≥2s(adjustable)
  canDMSSts : Inport
  canHeadDetn : Inport  Port=2
  canDistrctnLevel : Inport  Port=3
  canDistrctnQlty : Inport  Port=4
  PtDSGoodUnbeliv2MidDistractn : Inport  Port=5
  Compare To Constant : simulink/Logic and Bit Operations/Compare To Constant  relop===  const=2  OutDataTypeStr=boolean
  Compare To Constant1 : simulink/Logic and Bit Operations/Compare To Constant  relop===  const=1  OutDataTypeStr=boolean
  Compare To Constant2 : simulink/Logic and Bit Operations/Compare To Constant  relop===  const=2  OutDataTypeStr=boolean
  Compare To Constant4 : simulink/Logic and Bit Operations/Compare To Constant  relop=>=  const=85  OutDataTypeStr=boolean
  Compare To Constant8 : simulink/Logic and Bit Operations/Compare To Constant  relop=<=  const=100  OutDataTypeStr=boolean
  Data Type Conversion : DataTypeConversion  OutDataTypeStr=single
  Logical Operator : Logic  Inputs=5  AllPortsSameDT=off  OutDataTypeStr=boolean
  Relational Operator : RelationalOperator  OutDataTypeStr=boolean  RndMeth=Simplest
  counter : DiscreteIntegrator  ExternalReset=either  SampleTime=-1  LimitOutput=on  UpperSaturationLimit=10  LowerSaturationLimit=-10  ICPrevOutput=DiscIntNeverNeededParam  ICPrevScaledInput=DiscIntNeverNeededParam
  DSGoodUnbeliv2MidDistractn : Outport
  wires:
  Data Type Conversion/1 -> counter/1, counter/2
  counter/1 -> Relational Operator/1
  PtDSGoodUnbeliv2MidDistractn/1 -> Relational Operator/2
  Relational Operator/1 -> DSGoodUnbeliv2MidDistractn/1
  Compare To Constant8/1 -> Logical Operator/5
  Compare To Constant4/1 -> Logical Operator/4
  Compare To Constant2/1 -> Logical Operator/3
  Compare To Constant/1 -> Logical Operator/1
  Compare To Constant1/1 -> Logical Operator/2
  canDistrctnQlty/1 -> Compare To Constant4/1, Compare To Constant8/1
  Logical Operator/1 -> Data Type Conversion/1
  canDistrctnLevel/1 -> Compare To Constant2/1
  canHeadDetn/1 -> Compare To Constant1/1
  canDMSSts/1 -> Compare To Constant/1

== system Noh_Nofusion/Common1/Subsystem7/DS/DriverStsConditnJudge/DSGoodUnbeliv2MidDrowsnsJudge ==
  note: %Note
      | Conditions of drowsns state from Good∥Unbelievable to Middle as follow:
      | DMSSts_ACC is 0x02: Active
      | && HeadDetn is 0x01: Yes
      | && DrowsnsLevel_ACC is 0x2: Middle level Drowsiness
      | && DrowsnsQlty_ACC≥85%
      | && During time≥3s(adjustable)
  canDMSSts : Inport
  canHeadDetn : Inport  Port=2
  canDrowsnsLevel : Inport  Port=3
  PtDSGoodUnbeliv2MidDrowsns : Inport  Port=4
  Compare To Constant : simulink/Logic and Bit Operations/Compare To Constant  relop===  const=2  OutDataTypeStr=boolean
  Compare To Constant1 : simulink/Logic and Bit Operations/Compare To Constant  relop===  const=1  OutDataTypeStr=boolean
  Compare To Constant2 : simulink/Logic and Bit Operations/Compare To Constant  relop===  const=2  OutDataTypeStr=boolean
  Data Type Conversion : DataTypeConversion  OutDataTypeStr=single
  Logical Operator : Logic  Inputs=3  AllPortsSameDT=off  OutDataTypeStr=boolean
  Relational Operator : RelationalOperator  OutDataTypeStr=boolean  RndMeth=Simplest
  counter : DiscreteIntegrator  ExternalReset=either  SampleTime=-1  LimitOutput=on  UpperSaturationLimit=10  LowerSaturationLimit=-10  ICPrevOutput=DiscIntNeverNeededParam  ICPrevScaledInput=DiscIntNeverNeededParam
  DSGoodUnbeliv2MidDrowsns : Outport
  wires:
  Data Type Conversion/1 -> counter/1, counter/2
  PtDSGoodUnbeliv2MidDrowsns/1 -> Relational Operator/2
  canDMSSts/1 -> Compare To Constant/1
  canHeadDetn/1 -> Compare To Constant1/1
  canDrowsnsLevel/1 -> Compare To Constant2/1
  Logical Operator/1 -> Data Type Conversion/1
  counter/1 -> Relational Operator/1
  Relational Operator/1 -> DSGoodUnbeliv2MidDrowsns/1
  Compare To Constant1/1 -> Logical Operator/2
  Compare To Constant/1 -> Logical Operator/1
  Compare To Constant2/1 -> Logical Operator/3

== system Noh_Nofusion/Common1/Subsystem7/DS/DriverStsConditnJudge/DSHi1Hi22MidDistractnJudge ==
  note: %Note
      | Conditions of distraction state from High Level 1∥High Level 2 to Middle as follow:
      | DMSSts_ACC is 0x02: Active
      | && HeadDetn is 0x01: Yes
      | && DistrctnLevel_ACC is 0x02: Middle level distraction
      | && DistrctnQlty_ACC≥ 85%
      | && During time≥0.5s(adjustable)
  canDMSSts : Inport
  canHeadDetn : Inport  Port=2
  canDistrctnLevel : Inport  Port=3
  canDistrctnQlty : Inport  Port=4
  Compare To Constant : simulink/Logic and Bit Operations/Compare To Constant  relop===  const=2  OutDataTypeStr=boolean
  Compare To Constant1 : simulink/Logic and Bit Operations/Compare To Constant  relop===  const=1  OutDataTypeStr=boolean
  Compare To Constant2 : simulink/Logic and Bit Operations/Compare To Constant  relop===  const=2  OutDataTypeStr=boolean
  Compare To Constant4 : simulink/Logic and Bit Operations/Compare To Constant  relop=>=  const=85  OutDataTypeStr=boolean
  Compare To Constant5 : simulink/Logic and Bit Operations/Compare To Constant  relop=>=  const=0.5  OutDataTypeStr=boolean
  Compare To Constant8 : simulink/Logic and Bit Operations/Compare To Constant  relop=<=  const=100  OutDataTypeStr=boolean
  Data Type Conversion : DataTypeConversion  OutDataTypeStr=single
  Logical Operator : Logic  Inputs=5  AllPortsSameDT=off  OutDataTypeStr=boolean
  counter : DiscreteIntegrator  ExternalReset=either  SampleTime=-1  LimitOutput=on  UpperSaturationLimit=10  LowerSaturationLimit=-10  ICPrevOutput=DiscIntNeverNeededParam  ICPrevScaledInput=DiscIntNeverNeededParam
  DSHi1Hi22MidDistractn : Outport
  wires:
  Data Type Conversion/1 -> counter/1, counter/2
  canDMSSts/1 -> Compare To Constant/1
  canHeadDetn/1 -> Compare To Constant1/1
  canDistrctnLevel/1 -> Compare To Constant2/1
  Logical Operator/1 -> Data Type Conversion/1
  counter/1 -> Compare To Constant5/1
  canDistrctnQlty/1 -> Compare To Constant8/1, Compare To Constant4/1
  Compare To Constant1/1 -> Logical Operator/2
  Compare To Constant/1 -> Logical Operator/1
  Compare To Constant2/1 -> Logical Operator/3
  Compare To Constant4/1 -> Logical Operator/4
  Compare To Constant8/1 -> Logical Operator/5
  Compare To Constant5/1 -> DSHi1Hi22MidDistractn/1

== system Noh_Nofusion/Common1/Subsystem7/DS/DriverStsConditnJudge/DSHi1Hi22MidDrowsnsJudge ==
  note: %Note
      | Conditions of drowsns state from High Level 1∥High Level 2 to Middle as follow:
      | DMSSts_ACC is 0x02: Active
      | && HeadDetn is 0x01: Yes
      | && DrowsnsLevel_ACC is 0x2: Middle level Drowsiness
      | && DrowsnsQlty_ACC≥85%
      | && During time≥0.5s(adjustable)
  canDMSSts : Inport
  canHeadDetn : Inport  Port=2
  canDrowsnsLevel : Inport  Port=3
  Compare To Constant : simulink/Logic and Bit Operations/Compare To Constant  relop===  const=2  OutDataTypeStr=boolean
  Compare To Constant1 : simulink/Logic and Bit Operations/Compare To Constant  relop===  const=1  OutDataTypeStr=boolean
  Compare To Constant2 : simulink/Logic and Bit Operations/Compare To Constant  relop===  const=2  OutDataTypeStr=boolean
  Compare To Constant5 : simulink/Logic and Bit Operations/Compare To Constant  relop=>=  const=0.5  OutDataTypeStr=boolean
  Data Type Conversion : DataTypeConversion  OutDataTypeStr=single
  Logical Operator : Logic  Inputs=3  AllPortsSameDT=off  OutDataTypeStr=boolean
  counter : DiscreteIntegrator  ExternalReset=either  SampleTime=-1  LimitOutput=on  UpperSaturationLimit=10  LowerSaturationLimit=-10  ICPrevOutput=DiscIntNeverNeededParam  ICPrevScaledInput=DiscIntNeverNeededParam
  DSHi1Hi22MidDrowsns : Outport
  wires:
  Data Type Conversion/1 -> counter/1, counter/2
  Compare To Constant5/1 -> DSHi1Hi22MidDrowsns/1
  Compare To Constant2/1 -> Logical Operator/3
  Compare To Constant/1 -> Logical Operator/1
  Compare To Constant1/1 -> Logical Operator/2
  counter/1 -> Compare To Constant5/1
  Logical Operator/1 -> Data Type Conversion/1
  canDrowsnsLevel/1 -> Compare To Constant2/1
  canHeadDetn/1 -> Compare To Constant1/1
  canDMSSts/1 -> Compare To Constant/1

== system Noh_Nofusion/Common1/Subsystem7/DS/DriverStsConditnJudge/DSLow2MidDistractnJudge ==
  note: %Note
      | Conditions of distraction state from Low to Middle as follow:
      | DMSSts_ACC is 0x02: Active
      | && HeadDetn is 0x01: Yes
      | && DistrctnLevel_ACC is 0x02: Middle level distraction
      | && DistrctnQlty_ACC≥ 85%
      | && During time≥2s(adjustable)
  canDMSSts : Inport
  canHeadDetn : Inport  Port=2
  canDistrctnLevel : Inport  Port=3
  canDistrctnQlty : Inport  Port=4
  PtDSLow2MidDistractn : Inport  Port=5
  Compare To Constant : simulink/Logic and Bit Operations/Compare To Constant  relop===  const=2  OutDataTypeStr=boolean
  Compare To Constant1 : simulink/Logic and Bit Operations/Compare To Constant  relop===  const=1  OutDataTypeStr=boolean
  Compare To Constant2 : simulink/Logic and Bit Operations/Compare To Constant  relop===  const=2  OutDataTypeStr=boolean
  Compare To Constant4 : simulink/Logic and Bit Operations/Compare To Constant  relop=>=  const=85  OutDataTypeStr=boolean
  Compare To Constant8 : simulink/Logic and Bit Operations/Compare To Constant  relop=<=  const=100  OutDataTypeStr=boolean
  Data Type Conversion : DataTypeConversion  OutDataTypeStr=single
  Logical Operator : Logic  Inputs=5  AllPortsSameDT=off  OutDataTypeStr=boolean
  Relational Operator : RelationalOperator  OutDataTypeStr=boolean  RndMeth=Simplest
  counter : DiscreteIntegrator  ExternalReset=either  SampleTime=-1  LimitOutput=on  UpperSaturationLimit=10  LowerSaturationLimit=-10  ICPrevOutput=DiscIntNeverNeededParam  ICPrevScaledInput=DiscIntNeverNeededParam
  DSLow2MidDistractn : Outport
  wires:
  Data Type Conversion/1 -> counter/1, counter/2
  counter/1 -> Relational Operator/1
  PtDSLow2MidDistractn/1 -> Relational Operator/2
  canDMSSts/1 -> Compare To Constant/1
  canHeadDetn/1 -> Compare To Constant1/1
  canDistrctnLevel/1 -> Compare To Constant2/1
  Logical Operator/1 -> Data Type Conversion/1
  canDistrctnQlty/1 -> Compare To Constant8/1, Compare To Constant4/1
  Compare To Constant1/1 -> Logical Operator/2
  Compare To Constant/1 -> Logical Operator/1
  Compare To Constant2/1 -> Logical Operator/3
  Compare To Constant4/1 -> Logical Operator/4
  Compare To Constant8/1 -> Logical Operator/5
  Relational Operator/1 -> DSLow2MidDistractn/1

== system Noh_Nofusion/Common1/Subsystem7/DS/DriverStsConditnJudge/DSLow2MidDrowsnsJudge ==
  note: %Note
      | Conditions of drowsns state from Low to Middle as follow:
      | DMSSts_ACC is 0x02: Active
      | && HeadDetn is 0x01: Yes
      | && DrowsnsLevel_ACC is 0x2: Middle level Drowsiness
      | && DrowsnsQlty_ACC≥85%
      | && During time≥3s(adjustable)
  canDMSSts : Inport
  canHeadDetn : Inport  Port=2
  canDrowsnsLevel : Inport  Port=3
  PtDSLow2MidDrowsns : Inport  Port=4
  Compare To Constant : simulink/Logic and Bit Operations/Compare To Constant  relop===  const=2  OutDataTypeStr=boolean
  Compare To Constant1 : simulink/Logic and Bit Operations/Compare To Constant  relop===  const=1  OutDataTypeStr=boolean
  Compare To Constant2 : simulink/Logic and Bit Operations/Compare To Constant  relop===  const=2  OutDataTypeStr=boolean
  Data Type Conversion : DataTypeConversion  OutDataTypeStr=single
  Logical Operator : Logic  Inputs=3  AllPortsSameDT=off  OutDataTypeStr=boolean
  Relational Operator : RelationalOperator  OutDataTypeStr=boolean  RndMeth=Simplest
  counter : DiscreteIntegrator  ExternalReset=either  SampleTime=-1  LimitOutput=on  UpperSaturationLimit=10  LowerSaturationLimit=-10  ICPrevOutput=DiscIntNeverNeededParam  ICPrevScaledInput=DiscIntNeverNeededParam
  DSLow2MidDrowsns : Outport
  wires:
  Data Type Conversion/1 -> counter/1, counter/2
  PtDSLow2MidDrowsns/1 -> Relational Operator/2
  Relational Operator/1 -> DSLow2MidDrowsns/1
  Compare To Constant2/1 -> Logical Operator/3
  Compare To Constant/1 -> Logical Operator/1
  Compare To Constant1/1 -> Logical Operator/2
  counter/1 -> Relational Operator/1
  Logical Operator/1 -> Data Type Conversion/1
  canDrowsnsLevel/1 -> Compare To Constant2/1
  canHeadDetn/1 -> Compare To Constant1/1
  canDMSSts/1 -> Compare To Constant/1

== system Noh_Nofusion/Common1/Subsystem7/DS/DriverStsConditnJudge/DSMidHi1Hi22LowDistractnJudge ==
  note: %Note
      | Conditions of distraction state from Middle∥High Level 1∥High Level 2 to Low as follow:
      | DMSSts_ACC is 0x02: Active
      | && HeadDetn is 0x01: Yes
      | && DistrctnLevel_ACC is 0x01: Low level distraction
      | && DistrctnQlty_ACC≥ 85%
      | && During time≥0.5s(adjustable)
  canDMSSts : Inport
  canHeadDetn : Inport  Port=2
  canDistrctnLevel : Inport  Port=3
  canDistrctnQlty : Inport  Port=4
  Compare To Constant : simulink/Logic and Bit Operations/Compare To Constant  relop===  const=2  OutDataTypeStr=boolean
  Compare To Constant1 : simulink/Logic and Bit Operations/Compare To Constant  relop===  const=1  OutDataTypeStr=boolean
  Compare To Constant2 : simulink/Logic and Bit Operations/Compare To Constant  relop===  const=1  OutDataTypeStr=boolean
  Compare To Constant4 : simulink/Logic and Bit Operations/Compare To Constant  relop=>=  const=85  OutDataTypeStr=boolean
  Compare To Constant5 : simulink/Logic and Bit Operations/Compare To Constant  relop=>=  const=0.5  OutDataTypeStr=boolean
  Compare To Constant8 : simulink/Logic and Bit Operations/Compare To Constant  relop=<=  const=100  OutDataTypeStr=boolean
  Data Type Conversion : DataTypeConversion  OutDataTypeStr=single
  Logical Operator : Logic  Inputs=5  AllPortsSameDT=off  OutDataTypeStr=boolean
  counter : DiscreteIntegrator  ExternalReset=either  SampleTime=-1  LimitOutput=on  UpperSaturationLimit=10  LowerSaturationLimit=-10  ICPrevOutput=DiscIntNeverNeededParam  ICPrevScaledInput=DiscIntNeverNeededParam
  DSMidHi1Hi22LowDistractn : Outport
  wires:
  Data Type Conversion/1 -> counter/1, counter/2
  counter/1 -> Compare To Constant5/1
  canDMSSts/1 -> Compare To Constant/1
  canHeadDetn/1 -> Compare To Constant1/1
  canDistrctnLevel/1 -> Compare To Constant2/1
  Logical Operator/1 -> Data Type Conversion/1
  canDistrctnQlty/1 -> Compare To Constant8/1, Compare To Constant4/1
  Compare To Constant1/1 -> Logical Operator/2
  Compare To Constant/1 -> Logical Operator/1
  Compare To Constant2/1 -> Logical Operator/3
  Compare To Constant4/1 -> Logical Operator/4
  Compare To Constant8/1 -> Logical Operator/5
  Compare To Constant5/1 -> DSMidHi1Hi22LowDistractn/1

== system Noh_Nofusion/Common1/Subsystem7/DS/DriverStsConditnJudge/DSMidHi1Hi22LowDrowsnsJudge ==
  note: %Note
      | Conditions of drowsns state from Middle∥High Level 1∥High Level 2 to Low as follow:
      | DMSSts_ACC is 0x02: Active
      | && HeadDetn is 0x01: Yes
      | && DrowsnsLevel_ACC is 0x1: Low level Drowsiness
      | && DrowsnsQlty_ACC≥85%
      | && During time≥0.5s(adjustable)
  canDMSSts : Inport
  canHeadDetn : Inport  Port=2
  canDrowsnsLevel : Inport  Port=3
  Compare To Constant : simulink/Logic and Bit Operations/Compare To Constant  relop===  const=2  OutDataTypeStr=boolean
  Compare To Constant1 : simulink/Logic and Bit Operations/Compare To Constant  relop===  const=1  OutDataTypeStr=boolean
  Compare To Constant2 : simulink/Logic and Bit Operations/Compare To Constant  relop===  const=1  OutDataTypeStr=boolean
  Compare To Constant5 : simulink/Logic and Bit Operations/Compare To Constant  relop=>=  const=0.5  OutDataTypeStr=boolean
  Data Type Conversion : DataTypeConversion  OutDataTypeStr=single
  Logical Operator : Logic  Inputs=3  AllPortsSameDT=off  OutDataTypeStr=boolean
  counter : DiscreteIntegrator  ExternalReset=either  SampleTime=-1  LimitOutput=on  UpperSaturationLimit=10  LowerSaturationLimit=-10  ICPrevOutput=DiscIntNeverNeededParam  ICPrevScaledInput=DiscIntNeverNeededParam
  DSMidHi1Hi22LowDrowsns : Outport
  wires:
  Data Type Conversion/1 -> counter/1, counter/2
  counter/1 -> Compare To Constant5/1
  Compare To Constant5/1 -> DSMidHi1Hi22LowDrowsns/1
  Compare To Constant2/1 -> Logical Operator/3
  Compare To Constant/1 -> Logical Operator/1
  Compare To Constant1/1 -> Logical Operator/2
  Logical Operator/1 -> Data Type Conversion/1
  canDrowsnsLevel/1 -> Compare To Constant2/1
  canHeadDetn/1 -> Compare To Constant1/1
  canDMSSts/1 -> Compare To Constant/1
